simulink model "gm_sampleModel2001_1_sub"  (R2023a)
settings: Solver=VariableStepAuto  StartTime=0.0  StopTime=10.0  RelTol=1e-3
libraries: simulink x1
settings Model: Creator=user1  LastModifiedBy=user1
settings OptimizationCC: BlockReduction=off  ConditionallyExecuteInputs=off
settings DebuggingCC: InheritedTsInSrcMsg=none

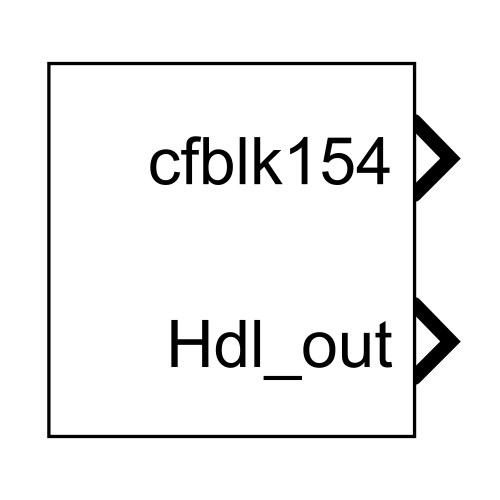
[thumbnail: Simulink's stored preview of the top-level diagram]
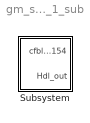
== system gm_sampleModel2001_1_sub ==
  Subsystem : Subsystem

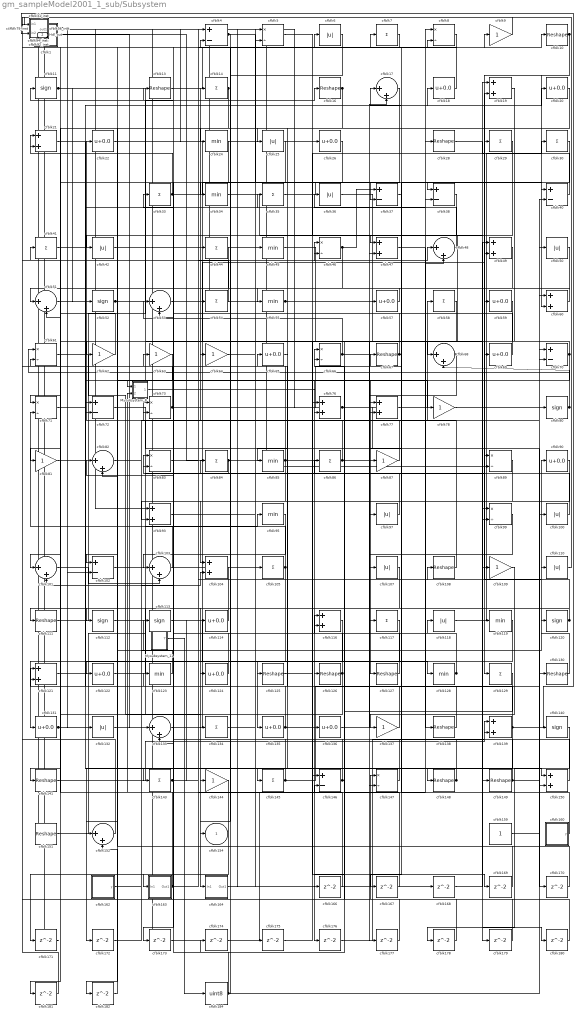
== system gm_sampleModel2001_1_sub/Subsystem ==
  Mysubsystem_11 : Subsystem
  Mysubsystem_8 : Subsystem
  cfblk1 : Subsystem  mask(Detect Fall Nonpositive){vinit=double(0), InputProcessing=Elements as channels (sample based), OutDataTypeStr=uint8}
      mask prompts: vinit "Simulink:masks:InitialCondition_MP"; InputProcessing "Simulink:masks:InputProcessing_MP"; OutDataTypeStr "Simulink:masks:OutputDataType_MP"
      mask help: Simulink:masks:DetectFallNonpositive_MD
      mask init:
      | InputProcessing = 'Elements as channels (sample based)';
      | OutDataTypeStr = 'uint8';
      | vinit = double(0);
      mask TypeOptions InputProcessing: Simulink:masks:ColumnsAsChannelsFrameBased | Simulink:masks:ElementsAsChannelsSampleBased
      mask TypeOptions OutDataTypeStr: Simulink:masks:uint8 | Simulink:masks:boolean
      mask Display: fprintf('U <= 0\n&  NOT\nU/z <= 0')
  cfblk{10,13,16,28,67,108,111,125..127,130,138,141,148..149,151} (16 alike) : Reshape
  cfblk{6,25,36,42,50,97,100,107,110,118,132} (11 alike) : Abs  OutDataTypeStr=uint8  SaturateOnIntegerOverflow=off
  cfblk{17,48,51,53,68,82,101,103,133,152} (10 alike) : Sum  Inputs=|++  OutDataTypeStr=uint8
  cfblk{4,37..38,40,70,72,102,146} (8 alike) : Sum  Inputs=+-  OutDataTypeStr=uint8
  cfblk{19,21,47,49,60,76..77,93,104,116,121,139,150} (13 alike) : Sum  OutDataTypeStr=uint8
  cfblk{7,14,29..30,33,35,41,44,54,58,84,86,105,117,129,134,143,145} (18 alike) : Sum  Inputs=+  OutDataTypeStr=uint8
  cfblk{9,62..64,78,81,87,109,137,144} (10 alike) : Gain  OutDataTypeStr=uint8
  cfblk{11,52,80,112..113,120,140} (7 alike) : Signum
  cfblk{18,20,22,26,57,59,65,69,90,114,122,124,131,135..136} (15 alike) : Bias  Bias=0.0  SaturateOnIntegerOverflow=off
  cfblk{24,34,45,55,85,95,119,123,128} (9 alike) : MinMax  OutDataTypeStr=uint8
  cfblk{5,8,46,61,66,71,73,83,89,99,147} (11 alike) : Product  Inputs=*/  OutDataTypeStr=uint8  RndMeth=Zero  SaturateOnIntegerOverflow=on
  cfblk153_inst : Subsystem
  cfblk159 : Constant  OutDataTypeStr=uint8  SampleTime=-1
  cfblk15_inst : Subsystem
  cfblk160 : Subsystem  mask(Counter Free-Running){NumBits=double(16), tsamp=double(-1)}
      mask prompts: NumBits "Simulink:masks:NumberOfBits_MP"; tsamp "Simulink:masks:SampleTime_MP"
      mask help: Simulink:masks:CounterFreeRunning_MD
  cfblk162 : Subsystem  mask(Counter Limited){uplimit=double(7), tsamp=double(-1)}
      mask prompts: uplimit "Simulink:masks:UpperLimit_MP"; tsamp "Simulink:masks:SampleTime_MP"
      mask help: Simulink:masks:CounterLimited_MD
      mask init:
      | nbits = double(8);
      | tsamp = double(-1);
      | uplimit = double(7);
  cfblk163 : Subsystem
  cfblk164 : Subsystem
  cfblk{166..182} (17 alike) : Delay  SampleTime=1
  cfblk184 : DataTypeConversion  OutDataTypeStr=uint8  SaturateOnIntegerOverflow=off  RndMeth=Floor
  cfblk2 : Constant  Value=0  OutDataTypeStr=uint8  SampleTime=1
  cfblk23_inst : Subsystem
  cfblk31_inst : Subsystem
  cfblk56_inst : Subsystem
  cfblk79_inst : Subsystem
  cfblk92_inst : Subsystem
  cfblk94_inst : Subsystem
  cfblk154 : Outport  OutDataTypeStr=uint8  SampleTime=1  VectorParamsAs1DForOutWhenUnconnected=off
  Hdl_out : Outport  Port=2  OutDataTypeStr=uint8  SampleTime=1
  wires:
  Mysubsystem_11/1(Y) -> cfblk184/1
  Mysubsystem_8/1(Out1) -> cfblk176/1
  cfblk1/1(Y) -> cfblk133/1
  cfblk10/1 -> cfblk60/2, cfblk129/1
  cfblk100/1 -> cfblk53/2
  cfblk101/1 -> cfblk103/2
  cfblk102/1 -> cfblk58/1
  cfblk103/1 -> cfblk71/2
  cfblk104/1 -> cfblk163/1(In1)
  cfblk105/1 -> cfblk164/1(In1), cfblk41/1
  cfblk107/1 -> cfblk144/1
  cfblk108/1 -> cfblk22/1
  cfblk109/1 -> cfblk137/1
  cfblk11/1 -> cfblk76/2, cfblk52/1, cfblk127/1
  cfblk110/1 -> cfblk31_inst/1(in1)
  cfblk111/1 -> cfblk16/1
  cfblk112/1 -> cfblk86/1
  cfblk113/1 -> cfblk126/1
  cfblk114/1 -> cfblk112/1
  cfblk116/1 -> cfblk131/1
  cfblk117/1 -> cfblk135/1
  cfblk118/1 -> cfblk30/1
  cfblk119/1 -> cfblk145/1
  cfblk120/1 -> cfblk19/2, cfblk111/1
  cfblk121/1 -> cfblk60/1
  cfblk122/1 -> cfblk8/1
  cfblk123/1 -> cfblk72/2
  cfblk124/1 -> cfblk33/1
  cfblk125/1 -> cfblk29/1
  cfblk126/1 -> cfblk82/1, cfblk141/1
  cfblk127/1 -> cfblk21/1
  cfblk128/1 -> cfblk118/1, cfblk63/1
  cfblk129/1 -> cfblk174/1
  cfblk13/1 -> cfblk6/1
  cfblk130/1 -> cfblk90/1
  cfblk131/1 -> cfblk40/2, cfblk95/1
  cfblk132/1 -> cfblk120/1
  cfblk133/1 -> cfblk49/2
  cfblk134/1 -> cfblk46/1
  cfblk135/1 -> cfblk17/2, cfblk121/1
  cfblk136/1 -> cfblk108/1
  cfblk137/1 -> cfblk65/1
  cfblk138/1 -> cfblk72/1
  cfblk139/1 -> cfblk56_inst/2(in2), cfblk173/1, cfblk172/1, cfblk123/1
  cfblk14/1 -> cfblk82/2, cfblk42/1, cfblk182/1
  cfblk140/1 -> cfblk178/1
  cfblk141/1 -> cfblk139/1
  cfblk143/1 -> cfblk150/1, cfblk114/1
  cfblk144/1 -> cfblk171/1
  cfblk145/1 -> cfblk70/2, cfblk121/2, cfblk113/1
  cfblk146/1 -> cfblk153_inst/1(in1), cfblk116/1
  cfblk147/1 -> cfblk84/1
  cfblk148/1 -> cfblk153_inst/2(in2), cfblk73/1
  cfblk149/1 -> cfblk130/1, cfblk101/2, cfblk66/1
  cfblk15_inst/1(out1) -> cfblk80/1
  cfblk150/1 -> cfblk7/1
  cfblk151/1 -> cfblk14/1
  cfblk152/1 -> cfblk92_inst/1(in1)
  cfblk153_inst/1(out1) -> cfblk93/1, cfblk45/1
  cfblk159/1 -> cfblk70/1
  cfblk16/1 -> cfblk51/2, cfblk85/1
  cfblk160/1(y) -> cfblk67/1
  cfblk162/1(y) -> cfblk104/2
  cfblk163/1(Out1) -> cfblk146/2, cfblk110/1, cfblk10/1, cfblk8/2, Mysubsystem_8/2(In2)
  cfblk164/1(Out1) -> cfblk5/2
  cfblk166/1 -> cfblk61/2
  cfblk167/1 -> cfblk66/2
  cfblk168/1 -> cfblk49/1
  cfblk169/1 -> cfblk4/2
  cfblk17/1 -> cfblk122/1
  cfblk170/1 -> cfblk92_inst/2(in2)
  cfblk171/1 -> cfblk1/1(U)
  cfblk172/1 -> cfblk38/2
  cfblk173/1 -> cfblk133/2
  cfblk174/1 -> cfblk48/2
  cfblk175/1 -> cfblk89/1
  cfblk176/1 -> cfblk139/2
  cfblk177/1 -> cfblk116/2
  cfblk178/1 -> cfblk15_inst/2(in2)
  cfblk179/1 -> cfblk56_inst/1(in1)
  cfblk18/1 -> cfblk5/1
  cfblk180/1 -> cfblk147/1
  cfblk181/1 -> cfblk79_inst/1(in1)
  cfblk182/1 -> cfblk152/2
  cfblk184/1 -> cfblk100/1, cfblk83/1, cfblk64/1
  cfblk19/1 -> cfblk69/1
  cfblk2/1 -> cfblk151/1, cfblk132/1
  cfblk20/1 -> cfblk25/1
  cfblk21/1 -> cfblk148/1
  cfblk22/1 -> cfblk99/1
  cfblk23_inst/1(out1) -> cfblk175/1
  cfblk24/1 -> cfblk143/1
  cfblk25/1 -> cfblk124/1
  cfblk26/1 -> cfblk181/1
  cfblk28/1 -> cfblk180/1
  cfblk29/1 -> cfblk68/1
  cfblk30/1 -> cfblk107/1
  cfblk31_inst/1(out1) -> cfblk168/1
  cfblk33/1 -> cfblk40/1, cfblk21/2
  cfblk34/1 -> cfblk109/1
  cfblk35/1 -> cfblk38/1
  cfblk36/1 -> cfblk119/1
  cfblk37/1 -> cfblk167/1
  cfblk38/1 -> cfblk152/1
  cfblk4/1 -> cfblk37/2, cfblk24/1
  cfblk40/1 -> cfblk19/1
  cfblk41/1 -> cfblk20/1
  cfblk42/1 -> cfblk146/1
  cfblk44/1 -> cfblk71/1
  cfblk45/1 -> cfblk177/1
  cfblk46/1 -> cfblk51/1, cfblk37/1
  cfblk47/1 -> cfblk138/1
  cfblk48/1 -> cfblk36/1
  cfblk49/1 -> cfblk81/1
  cfblk5/1 -> cfblk47/1
  cfblk50/1 -> cfblk77/1
  cfblk51/1 -> cfblk78/1
  cfblk52/1 -> cfblk28/1, cfblk136/1
  cfblk53/1 -> cfblk54/1
  cfblk54/1 -> cfblk15_inst/1(in1)
  cfblk55/1 -> cfblk149/1, cfblk99/2
  cfblk56_inst/1(out1) -> cfblk89/2
  cfblk57/1 -> cfblk55/1
  cfblk58/1 -> cfblk166/1
  cfblk59/1 -> cfblk101/1
  cfblk6/1 -> cfblk34/1
  cfblk60/1 -> cfblk59/1
  cfblk61/1 -> cfblk134/1
  cfblk62/1 -> cfblk23_inst/1(in1)
  cfblk63/1 -> cfblk102/1
  cfblk64/1 -> cfblk46/2
  cfblk65/1 -> cfblk125/1
  cfblk66/1 -> cfblk53/1, cfblk150/2
  cfblk67/1 -> cfblk17/1, cfblk13/1
  cfblk68/1 -> cfblk87/1, cfblk147/2
  cfblk69/1 -> cfblk11/1
  cfblk7/1 -> cfblk94_inst/2(in2)
  cfblk70/1 -> cfblk62/1, Mysubsystem_8/1(In1)
  cfblk71/1 -> cfblk128/1
  cfblk72/1 -> cfblk170/1
  cfblk73/1 -> cfblk47/2, cfblk31_inst/2(in2), cfblk169/1
  cfblk76/1 -> cfblk140/1, cfblk179/1
  cfblk77/1 -> cfblk9/1
  cfblk78/1 -> cfblk50/1
  cfblk79_inst/1(out1) -> cfblk26/1, cfblk105/1
  cfblk8/1 -> cfblk23_inst/2(in2)
  cfblk80/1 -> cfblk68/2, cfblk61/1
  cfblk81/1 -> cfblk35/1
  cfblk82/1 -> cfblk44/1
  cfblk83/1 -> cfblk48/1
  cfblk84/1 -> cfblk83/2, cfblk154/1
  cfblk85/1 -> cfblk93/2, cfblk79_inst/2(in2)
  cfblk86/1 -> cfblk77/2, cfblk73/2, Hdl_out/1
  cfblk87/1 -> cfblk4/1
  cfblk89/1 -> cfblk104/1
  cfblk9/1 -> cfblk94_inst/1(in1)
  cfblk90/1 -> cfblk97/1
  cfblk92_inst/1(out1) -> cfblk57/1
  cfblk93/1 -> cfblk18/1
  cfblk94_inst/1(out1) -> cfblk102/2
  cfblk95/1 -> cfblk103/1
  cfblk97/1 -> cfblk76/1
  cfblk99/1 -> cfblk117/1

== system gm_sampleModel2001_1_sub/Subsystem/Mysubsystem_11 ==
  cfblk161 : Subsystem  mask(Counter Free-Running){NumBits=double(16), tsamp=double(-1)}
      mask prompts: NumBits "Simulink:masks:NumberOfBits_MP"; tsamp "Simulink:masks:SampleTime_MP"
      mask help: Simulink:masks:CounterFreeRunning_MD
  cfblk185 : DataTypeConversion  OutDataTypeStr=uint8  SaturateOnIntegerOverflow=off  RndMeth=Floor
  cfblk3 : simulink/Logic and Bit Operations/Detect Change  vinit=0  OutDataTypeStr=boolean
      settings: LibrarySourceBlock=|
      | hdlsllib/Logic and Bit
      | Operations/Detect
      | Change
  Y : Outport  SampleTime=1
  wires:
  cfblk161/1(y) -> cfblk185/1
  cfblk185/1 -> cfblk3/1
  cfblk3/1 -> Y/1

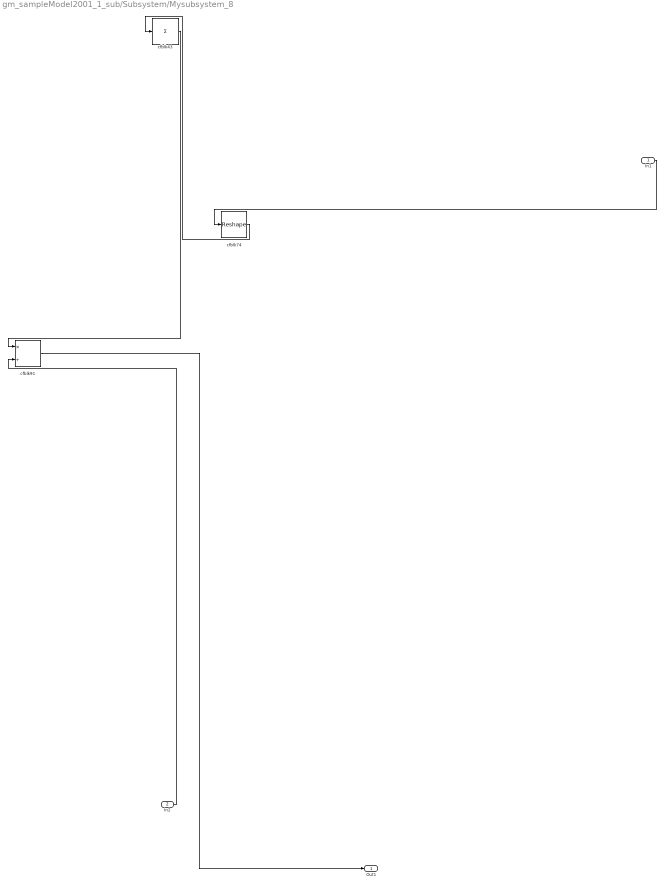
== system gm_sampleModel2001_1_sub/Subsystem/Mysubsystem_8 ==
  In1 : Inport  OutDataTypeStr=uint8  PortDimensions=1  SampleTime=1
  In2 : Inport  Port=2  OutDataTypeStr=uint8  PortDimensions=1  SampleTime=1
  cfblk43 : Sum  Inputs=+
  cfblk74 : Reshape
  cfblk91 : Product  Inputs=*/  RndMeth=Zero  SaturateOnIntegerOverflow=on
  Out1 : Outport  SampleTime=1
  wires:
  In1/1 -> cfblk74/1
  In2/1 -> cfblk91/2
  cfblk43/1 -> cfblk91/1
  cfblk74/1 -> cfblk43/1
  cfblk91/1 -> Out1/1

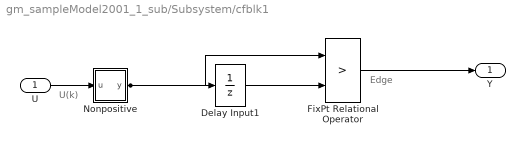
== system gm_sampleModel2001_1_sub/Subsystem/cfblk1 ==
  note: U(k)
  note: Edge
  U : Inport  OutDataTypeStr=uint8  SampleTime=1
  Delay Input1 : UnitDelay  Description=Store in Global RAM  DisableCoverage=on  InitialCondition=vinit  SampleTime=-1  HasFrameUpgradeWarning=on
  FixPt Relational Operator : RelationalOperator  Operator=>  OutDataTypeStr=fixdt(0, 8)  ZeroCross=off  InputSameDT=off
  Nonpositive : Subsystem  mask(Compare To Zero){relop=<=, OutDataTypeStr=boolean, ZeroCross=off}
      mask prompts: relop "Simulink:masks:Operator_MP"; OutDataTypeStr "Simulink:masks:OutputDataType_MP"; ZeroCross "Simulink:masks:EnableZerocrossingDetection_MP"
      mask help: Simulink:masks:CompareToZero_MD
      mask init:
      | OutDataTypeStr = 'boolean';
      | ZeroCross = 'off';
      | blkName = 'sampleModel2001_1_sub/Subsystem/cfblk1/Nonpositive';
      | relop = '<=';
      | setValue = 'boolean';
      mask TypeOptions relop: == | ~= | < | <= | >= | >
      mask TypeOptions OutDataTypeStr: Simulink:masks:uint8 | Simulink:masks:boolean
      mask Callback ZeroCross: sl('zeroCrossEnable', gcbh);
      mask Display: disp([relop,' 0'])
  Y : Outport  SampleTime=1
  wires:
  U/1 -> Nonpositive/1(u)
  Delay Input1/1 -> FixPt Relational Operator/2
  FixPt Relational Operator/1 -> Y/1
  Nonpositive/1(y) -> FixPt Relational Operator/1, Delay Input1/1

== system gm_sampleModel2001_1_sub/Subsystem/cfblk153_inst ==
  in1 : Inport  OutDataTypeStr=uint8  SampleTime=1
  in2 : Inport  Port=2  OutDataTypeStr=uint8  SampleTime=1
  mul_cfblk153_dotp_mulcomp : Product  Inputs=**  OutDataTypeStr=uint8  SampleTime=1
  out1 : Outport  OutDataTypeStr=uint8  SampleTime=1
  wires:
  in1/1 -> mul_cfblk153_dotp_mulcomp/1
  in2/1 -> mul_cfblk153_dotp_mulcomp/2
  mul_cfblk153_dotp_mulcomp/1 -> out1/1

== system gm_sampleModel2001_1_sub/Subsystem/cfblk15_inst ==
  in1 : Inport  OutDataTypeStr=uint8  SampleTime=1
  in2 : Inport  Port=2  OutDataTypeStr=uint8  SampleTime=1
  mul_cfblk15_dotp_mulcomp : Product  Inputs=**  OutDataTypeStr=uint8  SampleTime=1
  out1 : Outport  OutDataTypeStr=uint8  SampleTime=1
  wires:
  in1/1 -> mul_cfblk15_dotp_mulcomp/1
  in2/1 -> mul_cfblk15_dotp_mulcomp/2
  mul_cfblk15_dotp_mulcomp/1 -> out1/1

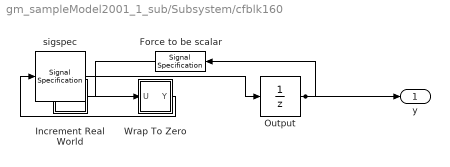
== system gm_sampleModel2001_1_sub/Subsystem/cfblk160 ==
  Force to be scalar : SignalSpecification  DisableCoverage=on  Dimensions=1
  Increment Real World : Subsystem  mask(Real World Value Increment){}
      mask help: Simulink:masks:RealWorldValueIncrement_MD
      mask Display: disp('V++')
  Output : UnitDelay  InitialCondition=0.0  SampleTime=tsamp  HasFrameUpgradeWarning=on
  Wrap To Zero : Subsystem  mask(Wrap To Zero){Threshold=double(65535)}
      mask prompts: Threshold "Simulink:masks:Threshold_MP"
      mask help: Simulink:masks:WrapToZero_MD
  sigspec : SignalSpecification  OutDataTypeStr=uint16  Dimensions=1
  y : Outport  SampleTime=1
  wires:
  Force to be scalar/1 -> Increment Real World/1(u)
  Increment Real World/1(y) -> Wrap To Zero/1(U)
  Output/1 -> Force to be scalar/1, y/1
  Wrap To Zero/1(Y) -> sigspec/1
  sigspec/1 -> Output/1

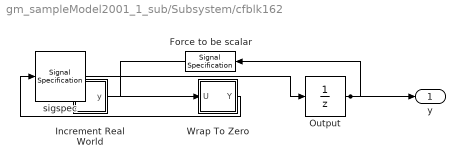
== system gm_sampleModel2001_1_sub/Subsystem/cfblk162 ==
  Force to be scalar : SignalSpecification  DisableCoverage=on  Dimensions=1
  Increment Real World : Subsystem  mask(Real World Value Increment){}
      mask help: Simulink:masks:RealWorldValueIncrement_MD
      mask Display: disp('V++')
  Output : UnitDelay  InitialCondition=0.0  SampleTime=tsamp  HasFrameUpgradeWarning=on
  Wrap To Zero : Subsystem  mask(Wrap To Zero){Threshold=double(7)}
      mask prompts: Threshold "Simulink:masks:Threshold_MP"
      mask help: Simulink:masks:WrapToZero_MD
  sigspec : SignalSpecification  OutDataTypeStr=uint8  Dimensions=1
  y : Outport  SampleTime=1
  wires:
  Force to be scalar/1 -> Increment Real World/1(u)
  Increment Real World/1(y) -> Wrap To Zero/1(U)
  Output/1 -> Force to be scalar/1, y/1
  Wrap To Zero/1(Y) -> sigspec/1
  sigspec/1 -> Output/1

== system gm_sampleModel2001_1_sub/Subsystem/cfblk163 ==
  In1 : Inport  OutDataTypeStr=uint8  PortDimensions=1  SampleTime=1
  Out1 : Outport  SampleTime=1
  wires:
  In1/1 -> Out1/1

== system gm_sampleModel2001_1_sub/Subsystem/cfblk164 ==
  In1 : Inport  OutDataTypeStr=uint8  PortDimensions=1  SampleTime=1
  Out1 : Outport  SampleTime=1
  wires:
  In1/1 -> Out1/1

== system gm_sampleModel2001_1_sub/Subsystem/cfblk23_inst ==
  in1 : Inport  OutDataTypeStr=uint8  SampleTime=1
  in2 : Inport  Port=2  OutDataTypeStr=uint8  SampleTime=1
  mul_cfblk23_dotp_mulcomp : Product  Inputs=**  OutDataTypeStr=uint8  SampleTime=1
  out1 : Outport  OutDataTypeStr=uint8  SampleTime=1
  wires:
  in1/1 -> mul_cfblk23_dotp_mulcomp/1
  in2/1 -> mul_cfblk23_dotp_mulcomp/2
  mul_cfblk23_dotp_mulcomp/1 -> out1/1

== system gm_sampleModel2001_1_sub/Subsystem/cfblk31_inst ==
  in1 : Inport  OutDataTypeStr=uint8  SampleTime=1
  in2 : Inport  Port=2  OutDataTypeStr=uint8  SampleTime=1
  mul_cfblk31_dotp_mulcomp : Product  Inputs=**  OutDataTypeStr=uint8  SampleTime=1
  out1 : Outport  OutDataTypeStr=uint8  SampleTime=1
  wires:
  in1/1 -> mul_cfblk31_dotp_mulcomp/1
  in2/1 -> mul_cfblk31_dotp_mulcomp/2
  mul_cfblk31_dotp_mulcomp/1 -> out1/1

== system gm_sampleModel2001_1_sub/Subsystem/cfblk56_inst ==
  in1 : Inport  OutDataTypeStr=uint8  SampleTime=1
  in2 : Inport  Port=2  OutDataTypeStr=uint8  SampleTime=1
  mul_cfblk56_dotp_mulcomp : Product  Inputs=**  OutDataTypeStr=uint8  SampleTime=1
  out1 : Outport  OutDataTypeStr=uint8  SampleTime=1
  wires:
  in1/1 -> mul_cfblk56_dotp_mulcomp/1
  in2/1 -> mul_cfblk56_dotp_mulcomp/2
  mul_cfblk56_dotp_mulcomp/1 -> out1/1

== system gm_sampleModel2001_1_sub/Subsystem/cfblk79_inst ==
  in1 : Inport  OutDataTypeStr=uint8  SampleTime=1
  in2 : Inport  Port=2  OutDataTypeStr=uint8  SampleTime=1
  mul_cfblk79_dotp_mulcomp : Product  Inputs=**  OutDataTypeStr=uint8  SampleTime=1
  out1 : Outport  OutDataTypeStr=uint8  SampleTime=1
  wires:
  in1/1 -> mul_cfblk79_dotp_mulcomp/1
  in2/1 -> mul_cfblk79_dotp_mulcomp/2
  mul_cfblk79_dotp_mulcomp/1 -> out1/1

== system gm_sampleModel2001_1_sub/Subsystem/cfblk92_inst ==
  in1 : Inport  OutDataTypeStr=uint8  SampleTime=1
  in2 : Inport  Port=2  OutDataTypeStr=uint8  SampleTime=1
  mul_cfblk92_dotp_mulcomp : Product  Inputs=**  OutDataTypeStr=uint8  SampleTime=1
  out1 : Outport  OutDataTypeStr=uint8  SampleTime=1
  wires:
  in1/1 -> mul_cfblk92_dotp_mulcomp/1
  in2/1 -> mul_cfblk92_dotp_mulcomp/2
  mul_cfblk92_dotp_mulcomp/1 -> out1/1

== system gm_sampleModel2001_1_sub/Subsystem/cfblk94_inst ==
  in1 : Inport  OutDataTypeStr=uint8  SampleTime=1
  in2 : Inport  Port=2  OutDataTypeStr=uint8  SampleTime=1
  mul_cfblk94_dotp_mulcomp : Product  Inputs=**  OutDataTypeStr=uint8  SampleTime=1
  out1 : Outport  OutDataTypeStr=uint8  SampleTime=1
  wires:
  in1/1 -> mul_cfblk94_dotp_mulcomp/1
  in2/1 -> mul_cfblk94_dotp_mulcomp/2
  mul_cfblk94_dotp_mulcomp/1 -> out1/1

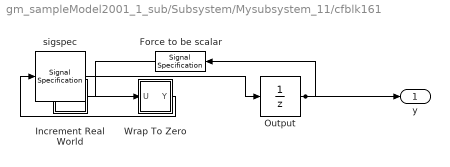
== system gm_sampleModel2001_1_sub/Subsystem/Mysubsystem_11/cfblk161 ==
  Force to be scalar : SignalSpecification  DisableCoverage=on  Dimensions=1
  Increment Real World : Subsystem  mask(Real World Value Increment){}
      mask help: Simulink:masks:RealWorldValueIncrement_MD
      mask Display: disp('V++')
  Output : UnitDelay  InitialCondition=0.0  SampleTime=tsamp  HasFrameUpgradeWarning=on
  Wrap To Zero : Subsystem  mask(Wrap To Zero){Threshold=double(65535)}
      mask prompts: Threshold "Simulink:masks:Threshold_MP"
      mask help: Simulink:masks:WrapToZero_MD
  sigspec : SignalSpecification  OutDataTypeStr=uint16  Dimensions=1
  y : Outport  SampleTime=1
  wires:
  Force to be scalar/1 -> Increment Real World/1(u)
  Increment Real World/1(y) -> Wrap To Zero/1(U)
  Output/1 -> Force to be scalar/1, y/1
  Wrap To Zero/1(Y) -> sigspec/1
  sigspec/1 -> Output/1

== system gm_sampleModel2001_1_sub/Subsystem/cfblk1/Nonpositive ==
  u : Inport  OutDataTypeStr=uint8  SampleTime=1
  Compare : RelationalOperator  Operator=<=  OutDataTypeStr=boolean  ZeroCross=off
  Constant : Constant  DisableCoverage=on  Value=0  OutDataTypeStr=Inherit: Inherit via back propagation  SampleTime=-1  PreserveConstantTs=on
  y : Outport  SampleTime=1
  wires:
  u/1 -> Compare/1
  Compare/1 -> y/1
  Constant/1 -> Compare/2

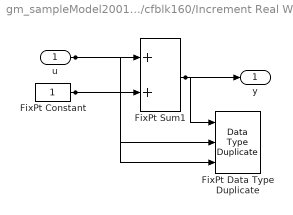
== system gm_sampleModel2001_1_sub/Subsystem/cfblk160/Increment Real World ==
  u : Inport  OutDataTypeStr=uint16  SampleTime=1
  FixPt Constant : Constant  DisableCoverage=on  OutDataTypeStr=Inherit: Inherit via back propagation  SampleTime=-1
  FixPt Data Type Duplicate : DataTypeDuplicate  DisableCoverage=on  NumInputPorts=3
  FixPt Sum1 : Sum  InputSameDT=on  OutDataTypeStr=Inherit: Inherit via back propagation  LockScale=on
  y : Outport  SampleTime=1
  wires:
  u/1 -> FixPt Sum1/1, FixPt Data Type Duplicate/2
  FixPt Constant/1 -> FixPt Sum1/2, FixPt Data Type Duplicate/3
  FixPt Sum1/1 -> FixPt Data Type Duplicate/1, y/1

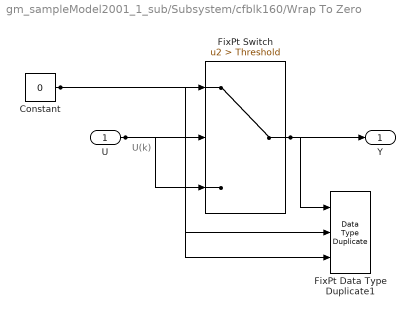
== system gm_sampleModel2001_1_sub/Subsystem/cfblk160/Wrap To Zero ==
  note: U(k)
  U : Inport  OutDataTypeStr=uint16  SampleTime=1
  Constant : Constant  DisableCoverage=on  Value=0  OutDataTypeStr=Inherit: Inherit via back propagation  SampleTime=-1
  FixPt Data Type Duplicate1 : DataTypeDuplicate  DisableCoverage=on  NumInputPorts=3
  FixPt Switch : Switch  Criteria=u2 > Threshold  Threshold=Threshold  OutDataTypeStr=Inherit: Inherit via back propagation  ZeroCross=off  SaturateOnIntegerOverflow=off  InputSameDT=off
  Y : Outport  SampleTime=1
  wires:
  U/1 -> FixPt Switch/3, FixPt Switch/2, FixPt Data Type Duplicate1/2
  Constant/1 -> FixPt Switch/1, FixPt Data Type Duplicate1/3
  FixPt Switch/1 -> FixPt Data Type Duplicate1/1, Y/1

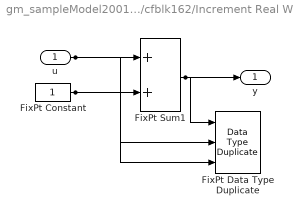
== system gm_sampleModel2001_1_sub/Subsystem/cfblk162/Increment Real World ==
  u : Inport  OutDataTypeStr=uint8  SampleTime=1
  FixPt Constant : Constant  DisableCoverage=on  OutDataTypeStr=Inherit: Inherit via back propagation  SampleTime=-1
  FixPt Data Type Duplicate : DataTypeDuplicate  DisableCoverage=on  NumInputPorts=3
  FixPt Sum1 : Sum  InputSameDT=on  OutDataTypeStr=Inherit: Inherit via back propagation  LockScale=on
  y : Outport  SampleTime=1
  wires:
  u/1 -> FixPt Sum1/1, FixPt Data Type Duplicate/2
  FixPt Constant/1 -> FixPt Sum1/2, FixPt Data Type Duplicate/3
  FixPt Sum1/1 -> FixPt Data Type Duplicate/1, y/1

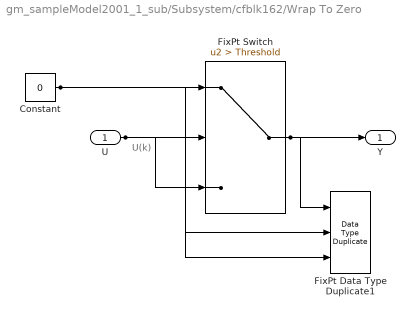
== system gm_sampleModel2001_1_sub/Subsystem/cfblk162/Wrap To Zero ==
  note: U(k)
  U : Inport  OutDataTypeStr=uint8  SampleTime=1
  Constant : Constant  DisableCoverage=on  Value=0  OutDataTypeStr=Inherit: Inherit via back propagation  SampleTime=-1
  FixPt Data Type Duplicate1 : DataTypeDuplicate  DisableCoverage=on  NumInputPorts=3
  FixPt Switch : Switch  Criteria=u2 > Threshold  Threshold=Threshold  OutDataTypeStr=Inherit: Inherit via back propagation  ZeroCross=off  SaturateOnIntegerOverflow=off  InputSameDT=off
  Y : Outport  SampleTime=1
  wires:
  U/1 -> FixPt Switch/3, FixPt Switch/2, FixPt Data Type Duplicate1/2
  Constant/1 -> FixPt Switch/1, FixPt Data Type Duplicate1/3
  FixPt Switch/1 -> FixPt Data Type Duplicate1/1, Y/1

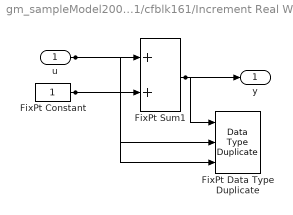
== system gm_sampleModel2001_1_sub/Subsystem/Mysubsystem_11/cfblk161/Increment Real World ==
  u : Inport  OutDataTypeStr=uint16  SampleTime=1
  FixPt Constant : Constant  DisableCoverage=on  OutDataTypeStr=Inherit: Inherit via back propagation  SampleTime=-1
  FixPt Data Type Duplicate : DataTypeDuplicate  DisableCoverage=on  NumInputPorts=3
  FixPt Sum1 : Sum  InputSameDT=on  OutDataTypeStr=Inherit: Inherit via back propagation  LockScale=on
  y : Outport  SampleTime=1
  wires:
  u/1 -> FixPt Sum1/1, FixPt Data Type Duplicate/2
  FixPt Constant/1 -> FixPt Sum1/2, FixPt Data Type Duplicate/3
  FixPt Sum1/1 -> FixPt Data Type Duplicate/1, y/1

== system gm_sampleModel2001_1_sub/Subsystem/Mysubsystem_11/cfblk161/Wrap To Zero ==
  note: U(k)
  U : Inport  OutDataTypeStr=uint16  SampleTime=1
  Constant : Constant  DisableCoverage=on  Value=0  OutDataTypeStr=Inherit: Inherit via back propagation  SampleTime=-1
  FixPt Data Type Duplicate1 : DataTypeDuplicate  DisableCoverage=on  NumInputPorts=3
  FixPt Switch : Switch  Criteria=u2 > Threshold  Threshold=Threshold  OutDataTypeStr=Inherit: Inherit via back propagation  ZeroCross=off  SaturateOnIntegerOverflow=off  InputSameDT=off
  Y : Outport  SampleTime=1
  wires:
  U/1 -> FixPt Switch/3, FixPt Switch/2, FixPt Data Type Duplicate1/2
  Constant/1 -> FixPt Switch/1, FixPt Data Type Duplicate1/3
  FixPt Switch/1 -> FixPt Data Type Duplicate1/1, Y/1
